simulink model "PR3_var15"  (R2020b)
settings: Solver=FixedStepAuto  StartTime=0.0  StopTime=5  FixedStep=0.01  RelTol=1e-3
settings Model: Creator=SIA  LastModifiedBy=SIA

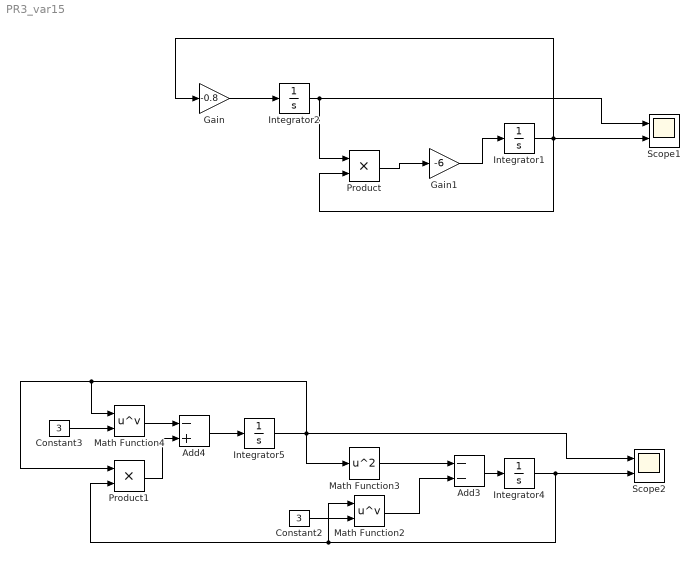
== system PR3_var15 ==
  Add3 : Sum  Inputs=--
  Add4 : Sum  Inputs=-+
  Constant2 : Constant  Value=3
  Constant3 : Constant  Value=3
  Gain : Gain  Gain=-0.8
  Gain1 : Gain  Gain=-6
  Integrator1 : Integrator  InitialCondition=2
  Integrator2 : Integrator  InitialCondition=2
  Integrator4 : Integrator  InitialCondition=1
  Integrator5 : Integrator  InitialCondition=1
  Math Function2 : Math  Operator=pow  SaturateOnIntegerOverflow=on
  Math Function3 : Math  Operator=square  SaturateOnIntegerOverflow=on
  Math Function4 : Math  Operator=pow  SaturateOnIntegerOverflow=on
  Product : Product
  Product1 : Product
  Scope1 : Scope  NumInputPorts=2
  Scope2 : Scope  NumInputPorts=2
  wires:
  Integrator5/1 -> Product1/1, Math Function4/1, Math Function3/1, Scope2/1
  Integrator4/1 -> Product1/2, Math Function2/1, Scope2/2
  Add3/1 -> Integrator4/1
  Constant2/1 -> Math Function2/2
  Math Function2/1 -> Add3/2
  Math Function3/1 -> Add3/1
  Add4/1 -> Integrator5/1
  Constant3/1 -> Math Function4/2
  Math Function4/1 -> Add4/1
  Product1/1 -> Add4/2
  Integrator1/1 -> Product/2, Gain/1, Scope1/2
  Gain/1 -> Integrator2/1
  Integrator2/1 -> Scope1/1, Product/1
  Gain1/1 -> Integrator1/1
  Product/1 -> Gain1/1
